simulink model "Ex2"  (Simulink 8.7)
settings: Solver=VariableStepAuto  StartTime=0.0  StopTime=10.0  RelTol=1e-3
settings Model: Creator=Perruci  LastModifiedBy=Perruci
settings DataIOCC: LimitDataPoints=off  SaveFormat=Dataset
settings DebuggingCC: UnderspecifiedInitializationDetection=Simplified  MergeDetectMultiDrivingBlocksExec=error
settings HardwareCC: ProdBitPerPointer=64  ProdLargestAtomicFloat=Float  ProdIntDivRoundTo=Zero  ProdEndianess=LittleEndian  ProdWordSize=64  ProdHWDeviceType=Intel->x86-64 (Windows64)
settings ModelReferenceCC: PropagateSignalLabelsOutOfModel=on
settings ConfigComp: CovModelRefEnable=off

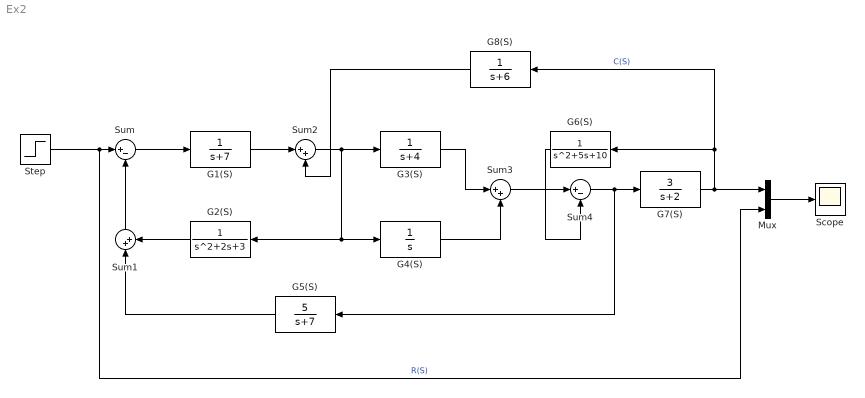
== system Ex2 ==
  G1(S) : TransferFcn  Denominator=[1 7]
  G2(S) : TransferFcn  Denominator=[1 2 3]
  G3(S) : TransferFcn  Denominator=[1 4]
  G4(S) : TransferFcn  Denominator=[1 0]
  G5(S) : TransferFcn  Numerator=[5]  Denominator=[1 7]
  G6(S) : TransferFcn  Denominator=[1 5 10]
  G7(S) : TransferFcn  Numerator=[3]  Denominator=[1 2]
  G8(S) : TransferFcn  Denominator=[1 6]
  Mux : Mux  Inputs=2
  Scope : Scope
  Step : Step  SampleTime=0
  Sum : Sum  Inputs=|+-
  Sum1 : Sum  Inputs=|++
  Sum2 : Sum  Inputs=|++
  Sum3 : Sum  Inputs=|++
  Sum4 : Sum  Inputs=|+-
  wires:
  Step/1 -> Mux/2, Sum/1  "R(S)"
  Sum/1 -> G1(S)/1
  Sum1/1 -> Sum/2
  G2(S)/1 -> Sum1/2
  Sum2/1 -> G3(S)/1, G2(S)/1, G4(S)/1
  G1(S)/1 -> Sum2/1
  G8(S)/1 -> Sum2/2
  Sum3/1 -> Sum4/1
  G3(S)/1 -> Sum3/1
  G4(S)/1 -> Sum3/2
  Sum4/1 -> G5(S)/1, G7(S)/1
  G7(S)/1 -> G8(S)/1, G6(S)/1, Mux/1  "C(S)"
  G6(S)/1 -> Sum4/2
  G5(S)/1 -> Sum1/1
  Mux/1 -> Scope/1
